simulink model "TurboShaftEngine_OpenLoop"  (R2023b)
settings: Solver=VariableStepAuto  StartTime=0.0  StopTime=1000  RelTol=1e-3
PreLoadFcn:
  | TurboShaftEngine_Params;
values from neighbouring files (symbols this model uses):
  combustor_volume = 0.001    [TurboShaftEngine_Params.m]
  flow_area = 0.002    [TurboShaftEngine_Params.m]
  shaft_inertia = 0.1    [TurboShaftEngine_Params.m]
libraries: fl_lib x34, nesl_utility x9, SimscapeFluids_lib x3, simulink x1, sdl_lib x1
(part 1 of 3)
settings Model: Creator=mprasad  LastModifiedBy=mprasad
settings SolverCC: MaxConsecutiveMinStep=2  AlgebraicLoopSolver=TrustRegion
settings DataIOCC: ReturnWorkspaceOutputs=off
settings DebuggingCC: UnconnectedInputMsg=warning  UnconnectedOutputMsg=warning  UnconnectedLineMsg=warning  PregeneratedLibrarySubsystemCodeDiagnostic=none  ArithmeticOperatorsInVariantConditions=warning
settings ModelReferenceCC: EnableRefExpFcnMdlSchedulingChecks=on
settings SFSimCC: SimUseLocalCustomCode=off  CustomCodeUndefinedFunction=UseInterfaceOnly
settings RTWCC: RTWUseLocalCustomCode=off  DLArmComputeVersion=19.05
settings CodeAppCC: StateflowObjectComments=on
settings SimscapeCC: SimscapeLogType=all  SimscapeLogSimulationStatistics=on  SimscapeLogName=simlog_TurboShaftEngine  SimscapeLogDataHistory=10000

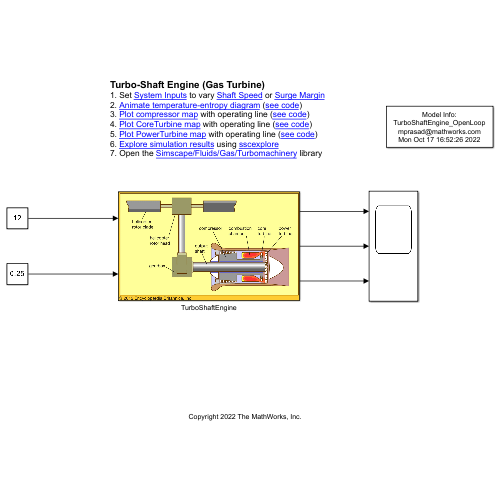
[thumbnail: Simulink's stored preview of the top-level diagram]
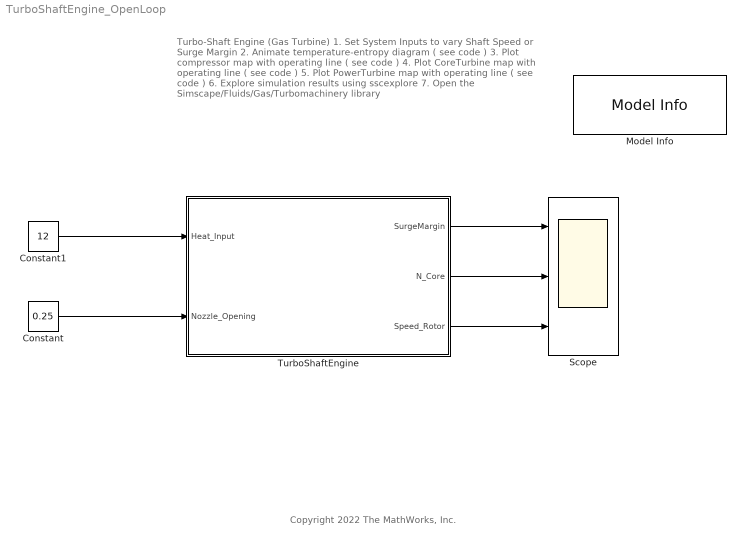
== system TurboShaftEngine_OpenLoop ==
  note: Turbo-Shaft Engine (Gas Turbine)
      | 1. Set System Inputs to vary Shaft Speed or Surge Margin
      | 2. Animate temperature-entropy diagram ( see code )
      | 3. Plot compressor map with operating line ( see code )
      | 4. Plot CoreTurbine map with operating line ( see code )
      | 5. Plot PowerTurbine map with operating line ( see code )
      | 6. Explore simulation results using sscexplore
      | 7. Open the Simscape/Fluids/Gas/Turbomachinery library
  note: Copyright 2022 The MathWorks, Inc.
  Constant : Constant  Value=0.25
  Constant1 : Constant  Value=12
  Model Info : simulink/Model-Wide Utilities/Model Info  Frame=on  DisplayStringWithTags=|  HorizontalTextAlignment=Center  LeftAlignmentValue=0.5
      | Model Info:
      | %<ModelName>
      | %<Creator>@mathworks.com
      | %<Created>
  Scope : Scope  NumInputPorts=3
  TurboShaftEngine : Subsystem
      mask Display: image('TurboShaftEngine.png'); % Use "Edit Image" on toolstrip to change.
  wires:
  Constant1/1 -> TurboShaftEngine/1(Heat_Input)
  Constant/1 -> TurboShaftEngine/2(Nozzle_Opening)
  TurboShaftEngine/1(SurgeMargin) -> Scope/1
  TurboShaftEngine/2(N_Core) -> Scope/2
  TurboShaftEngine/3(Speed_Rotor) -> Scope/3
